simulink model "GVCU_HIL_simscape"  (R2026a)
settings: Solver=ode3  StartTime=0  StopTime=10  FixedStep=0.001
model workspace (MAT data in the model file):
  CANoelibParameters : object (value not decoded)
values from neighbouring files (symbols this model uses):
  acc_pedal_data = pedal_data.accelerator_pedal_position_t0    [Init_Simscape_main.m]
  acc_pedal_time = pedal_data.t0    [Init_Simscape_main.m]
  brk_pedal_data = brake_pedal_data.shared_brakes_drvrBrkPedlPerc_t0    [Init_Simscape_main.m]
  brk_pedal_time = brake_pedal_data.t0    [Init_Simscape_main.m]
  cycle_len = zeros(1, num_cycles)    [Init_Simscape_main.m]
  cycle_speed_matrix = zeros(max_cycle_len, num_cycles)    [Init_Simscape_main.m]
  cycle_time_matrix = zeros(max_cycle_len, num_cycles)    [Init_Simscape_main.m]
  veh_speed_data = speed_data.shared_dynamicsVso_vehVelLgt_t0    [Init_Simscape_main.m]
  veh_speed_time = speed_data.t0    [Init_Simscape_main.m]
undefined symbols (not defined in the file or in its folder): Active, aero, AuxActive, bat, brake, config, environment, FL, FL_prs_voltage, FR, FR_prs_voltage, front, pos, powertrain, rear, RL, RL_prs_voltage, RR, RR_prs_voltage, tir, veh, VGetRawValueFlag, Voltage, VT2816_1_Ch1, VT2816_1_Ch2, VT2816_1_Ch3, VT2816_1_Ch4, VT2816_3_Ch13, VT2816_3_Ch14, VT7101_1_Out2, VTS, X, Y, Z
libraries: sm_lib x358, fl_lib x272, nesl_utility x193, canoelib x127, sdl_lib x36, autolibsharedcoupling x21, autolibcoupling x9, slpidlib x7, simulink x3, autolibshareddiff x3, autolibshared x3, autolibutils x1
(part 11 of 17)

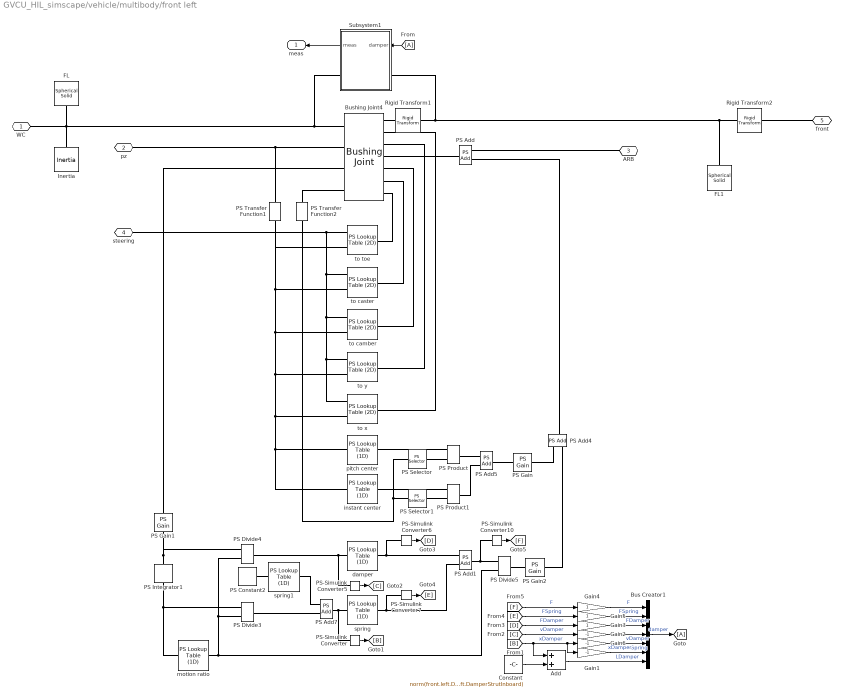
== system GVCU_HIL_simscape/vehicle/multibody/front left ==
  Add : Sum
  Bus Creator1 : BusCreator  Inputs=7
  Bushing Joint4 : sm_lib/Joints/Bushing Joint  JointMode=Normal  CompositeWrenchDir=FollowerOnBase  CompositeWrenchFrame=BaseFrame  SenseConstraintForce=off  SenseConstraintTorque=off  SenseTotalForce=on  SenseTotalTorque=off  PxPositionTargetSpecify=off  PxPositionTargetPriority=High  PxPositionTargetValue=0  PxPositionTargetValueUnits=m  PxVelocityTargetSpecify=off  PxVelocityTargetPriority=High  PxVelocityTargetValue=0  PxVelocityTargetValueUnits=m/s  PxEquilibriumPosition=0  PxEquilibriumPositionUnits=m  PxSpringStiffness=0  PxSpringStiffnessUnits=N/m  PxDampingCoefficient=0  PxDampingCoefficientUnits=N/(m/s)  PxLowerLimitSpecify=off  PxLowerLimitBound=-1  PxLowerLimitBoundUnits=m  PxLowerLimitStiffness=1e6  PxLowerLimitStiffnessUnits=N/m  PxLowerLimitDamping=1e3  PxLowerLimitDampingUnits=N/(m/s)  PxLowerLimitTransitionRegionWidth=1e-4  PxLowerLimitTransitionRegionWidthUnits=m  PxUpperLimitSpecify=off  PxUpperLimitBound=1  PxUpperLimitBoundUnits=m  PxUpperLimitStiffness=1e6  PxUpperLimitStiffnessUnits=N/m  PxUpperLimitDamping=1e3  PxUpperLimitDampingUnits=N/(m/s)  PxUpperLimitTransitionRegionWidth=1e-4  PxUpperLimitTransitionRegionWidthUnits=m  PxTorqueActuationMode=ComputedTorque  PxMotionActuationMode=InputMotion  PxSensePosition=off  PxSenseVelocity=off  PxSenseAcceleration=off  PxSenseTorqueForce=off  PxSenseLowerLimitTorqueForce=off  PxSenseUpperLimitTorqueForce=off  PyPositionTargetSpecify=off  PyPositionTargetPriority=High  PyPositionTargetValue=0  PyPositionTargetValueUnits=m  PyVelocityTargetSpecify=off  PyVelocityTargetPriority=High  PyVelocityTargetValue=0  PyVelocityTargetValueUnits=m/s  PyEquilibriumPosition=0  PyEquilibriumPositionUnits=m  PySpringStiffness=0  PySpringStiffnessUnits=N/m  PyDampingCoefficient=0  PyDampingCoefficientUnits=N/(m/s)  PyLowerLimitSpecify=off  PyLowerLimitBound=-1  PyLowerLimitBoundUnits=m  PyLowerLimitStiffness=1e6  PyLowerLimitStiffnessUnits=N/m  PyLowerLimitDamping=1e3  PyLowerLimitDampingUnits=N/(m/s)  PyLowerLimitTransitionRegionWidth=1e-4  PyLowerLimitTransitionRegionWidthUnits=m  PyUpperLimitSpecify=off  PyUpperLimitBound=1  PyUpperLimitBoundUnits=m  PyUpperLimitStiffness=1e6  PyUpperLimitStiffnessUnits=N/m  PyUpperLimitDamping=1e3  PyUpperLimitDampingUnits=N/(m/s)  PyUpperLimitTransitionRegionWidth=1e-4  PyUpperLimitTransitionRegionWidthUnits=m  PyTorqueActuationMode=ComputedTorque  PyMotionActuationMode=InputMotion  PySensePosition=off  PySenseVelocity=off  PySenseAcceleration=off  PySenseTorqueForce=off  PySenseLowerLimitTorqueForce=off  PySenseUpperLimitTorqueForce=off  PzPositionTargetSpecify=off  PzPositionTargetPriority=High  PzPositionTargetValue=0  PzPositionTargetValueUnits=m  PzVelocityTargetSpecify=off  PzVelocityTargetPriority=High  PzVelocityTargetValue=0  PzVelocityTargetValueUnits=m/s  PzEquilibriumPosition=0  PzEquilibriumPositionUnits=m  PzSpringStiffness=0  PzSpringStiffnessUnits=N/m  PzDampingCoefficient=0  PzDampingCoefficientUnits=N/(m/s)  PzLowerLimitSpecify=off  PzLowerLimitBound=-1  PzLowerLimitBoundUnits=m  PzLowerLimitStiffness=1e6  PzLowerLimitStiffnessUnits=N/m  PzLowerLimitDamping=1e3  PzLowerLimitDampingUnits=N/(m/s)  PzLowerLimitTransitionRegionWidth=1e-4  PzLowerLimitTransitionRegionWidthUnits=m  PzUpperLimitSpecify=off  PzUpperLimitBound=1  PzUpperLimitBoundUnits=m  PzUpperLimitStiffness=1e6  PzUpperLimitStiffnessUnits=N/m  PzUpperLimitDamping=1e3  PzUpperLimitDampingUnits=N/(m/s)  PzUpperLimitTransitionRegionWidth=1e-4  PzUpperLimitTransitionRegionWidthUnits=m  PzTorqueActuationMode=InputTorque  PzMotionActuationMode=ComputedMotion  PzSensePosition=on  PzSenseVelocity=on  PzSenseAcceleration=off  PzSenseTorqueForce=off  PzSenseLowerLimitTorqueForce=off  PzSenseUpperLimitTorqueForce=off  RxPositionTargetSpecify=off  RxPositionTargetPriority=High  RxPositionTargetValue=0  RxPositionTargetValueUnits=deg  RxVelocityTargetSpecify=off  RxVelocityTargetPriority=High  RxVelocityTargetValue=0  RxVelocityTargetValueUnits=deg/s  RxEquilibriumPosition=0  RxEquilibriumPositionUnits=deg  RxSpringStiffness=0  RxSpringStiffnessUnits=N*m/deg  RxDampingCoefficient=0  RxDampingCoefficientUnits=N*m/(deg/s)  RxLowerLimitSpecify=off  RxLowerLimitBound=-90  RxLowerLimitBoundUnits=deg  RxLowerLimitStiffness=1e4  RxLowerLimitStiffnessUnits=N*m/deg  RxLowerLimitDamping=10  RxLowerLimitDampingUnits=N*m/(deg/s)  RxLowerLimitTransitionRegionWidth=0.1  RxLowerLimitTransitionRegionWidthUnits=deg  RxUpperLimitSpecify=off  RxUpperLimitBound=90  RxUpperLimitBoundUnits=deg  RxUpperLimitStiffness=1e4  RxUpperLimitStiffnessUnits=N*m/deg  RxUpperLimitDamping=10  RxUpperLimitDampingUnits=N*m/(deg/s)  RxUpperLimitTransitionRegionWidth=0.1  RxUpperLimitTransitionRegionWidthUnits=deg  RxTorqueActuationMode=ComputedTorque  RxMotionActuationMode=InputMotion  RxSensePosition=off  RxSenseVelocity=off  RxSenseAcceleration=off  RxSenseTorqueForce=off  RxSenseLowerLimitTorqueForce=off  RxSenseUpperLimitTorqueForce=off  RyPositionTargetSpecify=off  RyPositionTargetPriority=High  RyPositionTargetValue=0  RyPositionTargetValueUnits=deg  RyVelocityTargetSpecify=off  RyVelocityTargetPriority=High  RyVelocityTargetValue=0  RyVelocityTargetValueUnits=deg/s  RyEquilibriumPosition=0  RyEquilibriumPositionUnits=deg  RySpringStiffness=0  RySpringStiffnessUnits=N*m/deg  RyDampingCoefficient=0  RyDampingCoefficientUnits=N*m/(deg/s)  RyLowerLimitSpecify=off  RyLowerLimitBound=-90  RyLowerLimitBoundUnits=deg  RyLowerLimitStiffness=1e4  RyLowerLimitStiffnessUnits=N*m/deg  RyLowerLimitDamping=10  RyLowerLimitDampingUnits=N*m/(deg/s)  RyLowerLimitTransitionRegionWidth=0.1  RyLowerLimitTransitionRegionWidthUnits=deg  RyUpperLimitSpecify=off  RyUpperLimitBound=90  RyUpperLimitBoundUnits=deg  RyUpperLimitStiffness=1e4  RyUpperLimitStiffnessUnits=N*m/deg  RyUpperLimitDamping=10  RyUpperLimitDampingUnits=N*m/(deg/s)  RyUpperLimitTransitionRegionWidth=0.1  RyUpperLimitTransitionRegionWidthUnits=deg  RyTorqueActuationMode=ComputedTorque  RyMotionActuationMode=InputMotion  RySensePosition=off  RySenseVelocity=off  RySenseAcceleration=off  RySenseTorqueForce=off  RySenseLowerLimitTorqueForce=off  RySenseUpperLimitTorqueForce=off  RzPositionTargetSpecify=off  RzPositionTargetPriority=High  RzPositionTargetValue=0  RzPositionTargetValueUnits=deg  RzVelocityTargetSpecify=off  RzVelocityTargetPriority=High  RzVelocityTargetValue=0  RzVelocityTargetValueUnits=deg/s  RzEquilibriumPosition=0  RzEquilibriumPositionUnits=deg  RzSpringStiffness=0  RzSpringStiffnessUnits=N*m/deg  RzDampingCoefficient=0  RzDampingCoefficientUnits=N*m/(deg/s)  RzLowerLimitSpecify=off  RzLowerLimitBound=-90  RzLowerLimitBoundUnits=deg  RzLowerLimitStiffness=1e4  RzLowerLimitStiffnessUnits=N*m/deg  RzLowerLimitDamping=10  RzLowerLimitDampingUnits=N*m/(deg/s)  RzLowerLimitTransitionRegionWidth=0.1  RzLowerLimitTransitionRegionWidthUnits=deg  RzUpperLimitSpecify=off  RzUpperLimitBound=90  RzUpperLimitBoundUnits=deg  RzUpperLimitStiffness=1e4  RzUpperLimitStiffnessUnits=N*m/deg  RzUpperLimitDamping=10  RzUpperLimitDampingUnits=N*m/(deg/s)  RzUpperLimitTransitionRegionWidth=0.1  RzUpperLimitTransitionRegionWidthUnits=deg  RzTorqueActuationMode=ComputedTorque  RzMotionActuationMode=InputMotion  RzSensePosition=off  RzSenseVelocity=off  RzSenseAcceleration=off  RzSenseTorqueForce=off  RzSenseLowerLimitTorqueForce=off  RzSenseUpperLimitTorqueForce=off
  Constant : Constant  Value=norm(front.left.DamperStrutOutboard-front.left.DamperStrutInboard)
  FL : sm_lib/Body Elements/Spherical Solid  SphereRadius=vis.joint.r  SphereRadiusUnits=m  ExportEntireGeometry=off  InertiaType=PointMass  BasedOnType=Density  Density=0  DensityUnits=kg/m^3  Mass=0  MassUnits=kg  CenterOfMass=[0 0 0]  CenterOfMassUnits=m  MomentsOfInertia=[1 1 1]  MomentsOfInertiaUnits=kg*m^2  ProductsOfInertia=[0 0 0]  ProductsOfInertiaUnits=kg*m^2  GraphicType=FromGeometry  MarkerShape=Sphere  MarkerSize=10  GraphicVisPropType=SimpleVisualProperties  GraphicDiffuseColor=vis.joint.color  GraphicOpacity=1  GraphicSpecularColor=[0.5 0.5 0.5 1.0]  GraphicAmbientColor=[0.15 0.15 0.15 1.0]  GraphicEmissiveColor=[0.0 0.0 0.0 1.0]  GraphicShininess=75  DoExposeReferenceFrame=on  SerializedFrames=<Frames/>
  FL1 : sm_lib/Body Elements/Spherical Solid  SphereRadius=vis.joint.r  SphereRadiusUnits=m  ExportEntireGeometry=off  InertiaType=PointMass  BasedOnType=Density  Density=0  DensityUnits=kg/m^3  Mass=0  MassUnits=kg  CenterOfMass=[0 0 0]  CenterOfMassUnits=m  MomentsOfInertia=[1 1 1]  MomentsOfInertiaUnits=kg*m^2  ProductsOfInertia=[0 0 0]  ProductsOfInertiaUnits=kg*m^2  GraphicType=FromGeometry  MarkerShape=Sphere  MarkerSize=10  GraphicVisPropType=SimpleVisualProperties  GraphicDiffuseColor=vis.joint.color  GraphicOpacity=1  GraphicSpecularColor=[0.5 0.5 0.5 1.0]  GraphicAmbientColor=[0.15 0.15 0.15 1.0]  GraphicEmissiveColor=[0.0 0.0 0.0 1.0]  GraphicShininess=75  DoExposeReferenceFrame=on  SerializedFrames=<Frames/>
  From : From
  Gain1 : Gain  Gain=-1
  Gain2 : Gain  Gain=-1
  Gain3 : Gain
  Gain4 : Gain
  Gain5 : Gain
  Gain6 : Gain  Gain=-1
  Goto : Goto
  Inertia : sm_lib/Body Elements/Inertia  InertiaType=PointMass  Mass=front.unsprung_mass  MassUnits=kg  CenterOfMass=[0 0 0]  CenterOfMassUnits=m  MomentsOfInertia=[1 1 1]  MomentsOfInertiaUnits=kg*m^2  ProductsOfInertia=[0 0 0]  ProductsOfInertiaUnits=kg*m^2  GraphicType=None  MarkerShape=Inertia  MarkerSize=20  GraphicVisPropType=SimpleVisualProperties  GraphicDiffuseColor=[0.5 0.5 0.5]  GraphicOpacity=1  GraphicSpecularColor=[0.5 0.5 0.5 1.0]  GraphicAmbientColor=[0.15 0.15 0.15 1.0]  GraphicEmissiveColor=[0.0 0.0 0.0 1.0]  GraphicShininess=75
  PS Add{,1,4..5,7} (5 alike) : fl_lib/Physical Signals/Functions/PS Add
  PS Constant2 : fl_lib/Physical Signals/Sources/PS Constant  constant=front.spring.preload N
  PS Divide3 : fl_lib/Physical Signals/Functions/PS Divide
  PS Divide4 : fl_lib/Physical Signals/Functions/PS Divide
  PS Divide5 : fl_lib/Physical Signals/Functions/PS Divide
  PS Gain : fl_lib/Physical Signals/Functions/PS Gain  gain=1
  PS Gain1 : fl_lib/Physical Signals/Functions/PS Gain  gain=1
  PS Gain2 : fl_lib/Physical Signals/Functions/PS Gain  gain=-1
  PS Integrator1 : fl_lib/Physical Signals/Linear Operators/PS Integrator  reset_method=foundation.enum.IntegratorResetSpec.None  initial_condition_spec=foundation.enum.IntegratorICSpec.Internal  saturation_spec=foundation.enum.IntegratorSaturationSpec.None  saturation_source_spec=foundation.enum.IntegratorSaturationSourceSpec.Internal  x0=0 m  xu=inf s  xl=-inf s
  PS Product : fl_lib/Physical Signals/Functions/PS Product
  PS Product1 : fl_lib/Physical Signals/Functions/PS Product
  PS Selector : fl_lib/Physical Signals/Nonlinear Operators/PS Selector  ix=1
  PS Selector1 : fl_lib/Physical Signals/Nonlinear Operators/PS Selector  ix=2
  PS Transfer Function1 : fl_lib/Physical Signals/Linear Operators/PS Transfer Function  transfer_function_type=foundation.enum.transfer_function_type.lag  T=0.001 s  T1=2 s  T2=1 s  reset_method=foundation.enum.IntegratorResetSpec.None  initial_condition_spec=foundation.enum.IntegratorICSpec.Internal  y0=0 m
  PS Transfer Function2 : fl_lib/Physical Signals/Linear Operators/PS Transfer Function  transfer_function_type=foundation.enum.transfer_function_type.lag  T=0.001 s  T1=2 s  T2=1 s  reset_method=foundation.enum.IntegratorResetSpec.None  initial_condition_spec=foundation.enum.IntegratorICSpec.Internal  y0=0 N
  PS-Simulink Converter{,5..7,10} (5 alike) : nesl_utility/PS-Simulink Converter  PhysicalDomain=network_engine_domain  SubClassName=ps_output  LeftPortType=input  RightPortType=output  PseudoPeriodic=off  Frequencies=[]  VectorFormat=inherit  Unit=inherit  AffineConversion=off
  Rigid Transform1 : sm_lib/Frames and Transforms/Rigid Transform  RotationMethod=RotationSequence  FollAlignAxisA=+X  BaseAlignAxisA=+Y  FollAlignAxisB=+Y  BaseAlignAxisB=+Z  RotationStandardAxis=+X  RotationAngle=0.5  RotationAngleUnits=deg  RotationArbitraryAxis=[0 0 1]  RotationSequenceAxes=FollowerAxes  RotationSequence=XYZ  RotationSequenceAngles=[-front.wheel.camber 0 front.wheel.toe]  RotationSequenceAnglesUnits=deg  RotationMatrix=[1 0 0;0 1 0;0 0 1]  Quaternion=[1 0 0 0]  TranslationMethod=None  TranslationCartesianOffset=[0 0 0]  TranslationCartesianOffsetUnits=m  TranslationStandardAxis=+Z  TranslationStandardOffset=0  TranslationStandardOffsetUnits=m  TranslationROffset=0  TranslationROffsetUnits=m  TranslationThetaOffset=0  TranslationThetaOffsetUnits=deg  TranslationZOffset=0  TranslationZOffsetUnits=m
  Rigid Transform2 : sm_lib/Frames and Transforms/Rigid Transform  RotationMethod=None  FollAlignAxisA=+X  BaseAlignAxisA=+Y  FollAlignAxisB=+Y  BaseAlignAxisB=+Z  RotationStandardAxis=+Z  RotationAngle=0  RotationAngleUnits=deg  RotationArbitraryAxis=[0 0 1]  RotationSequenceAxes=FollowerAxes  RotationSequence=XYX  RotationSequenceAngles=[0 0 0]  RotationSequenceAnglesUnits=deg  RotationMatrix=[1 0 0;0 1 0;0 0 1]  Quaternion=[1 0 0 0]  TranslationMethod=Cartesian  TranslationCartesianOffset=front.left.WheelC  TranslationCartesianOffsetUnits=m  TranslationStandardAxis=+Z  TranslationStandardOffset=0  TranslationStandardOffsetUnits=m  TranslationROffset=0  TranslationROffsetUnits=m  TranslationThetaOffset=0  TranslationThetaOffsetUnits=deg  TranslationZOffset=0  TranslationZOffsetUnits=m
  Subsystem1 : Subsystem
  damper : fl_lib/Physical Signals/Lookup Tables/PS Lookup Table (1D)  x=front.damper.v m/s  f=front.damper.N N  interp_method=simscape.enum.interpolation.linear  extrap_method=simscape.enum.extrapolation.linear
  instant center : fl_lib/Physical Signals/Lookup Tables/PS Lookup Table (1D)  x=front.z_bp m  f=tan(-front.IC_alpha)  interp_method=simscape.enum.interpolation.linear  extrap_method=simscape.enum.extrapolation.linear
  motion ratio : fl_lib/Physical Signals/Lookup Tables/PS Lookup Table (1D)  x=front.z_bp m  f=front.spring.mr_bp  interp_method=simscape.enum.interpolation.linear  extrap_method=simscape.enum.extrapolation.nearest
  pitch center : fl_lib/Physical Signals/Lookup Tables/PS Lookup Table (1D)  x=front.z_bp m  f=tan(-front.PC_alpha)  interp_method=simscape.enum.interpolation.linear  extrap_method=simscape.enum.extrapolation.linear
  spring : fl_lib/Physical Signals/Lookup Tables/PS Lookup Table (1D)  x=front.spring.l m  f=front.spring.N N  interp_method=simscape.enum.interpolation.linear  extrap_method=simscape.enum.extrapolation.linear
  spring1 : fl_lib/Physical Signals/Lookup Tables/PS Lookup Table (1D)  x=front.spring.N(2:end) N  f=front.spring.l(2:end) m  interp_method=simscape.enum.interpolation.linear  extrap_method=simscape.enum.extrapolation.linear
  to camber : fl_lib/Physical Signals/Lookup Tables/PS Lookup Table (2D)  x1=front.tierod_bp m  x2=front.z_bp m  f=front.left.camber_bp rad  interp_method=simscape.enum.interpolation.linear  extrap_method=simscape.enum.extrapolation.linear
  to caster : fl_lib/Physical Signals/Lookup Tables/PS Lookup Table (2D)  x1=front.tierod_bp m  x2=front.z_bp m  f=front.left.caster_bp rad  interp_method=simscape.enum.interpolation.linear  extrap_method=simscape.enum.extrapolation.linear
  to toe : fl_lib/Physical Signals/Lookup Tables/PS Lookup Table (2D)  x1=front.tierod_bp m  x2=front.z_bp m  f=front.left.toe_bp rad  interp_method=simscape.enum.interpolation.linear  extrap_method=simscape.enum.extrapolation.linear
  to x : fl_lib/Physical Signals/Lookup Tables/PS Lookup Table (2D)  x1=front.tierod_bp m  x2=front.z_bp m  f=front.left.x_bp m  interp_method=simscape.enum.interpolation.linear  extrap_method=simscape.enum.extrapolation.linear
  to y : fl_lib/Physical Signals/Lookup Tables/PS Lookup Table (2D)  x1=front.tierod_bp m  x2=front.z_bp m  f=front.left.y_bp m  interp_method=simscape.enum.interpolation.linear  extrap_method=simscape.enum.extrapolation.linear
  WC : PMIOPort  Side=Left
  pz : PMIOPort  Port=2  Side=Right
  ARB : PMIOPort  Port=3  Side=Right
  steering : PMIOPort  Port=4  Side=Right
  front : PMIOPort  Port=5  Side=Right
  meas : Outport
  wires:
  Subsystem1/1(meas) -> meas/1
  Add/1 -> Bus Creator1/7  "LDamper"
  Bus Creator1/1 -> Goto/1  "damper"
  [E] -> Gain5/1  "FSpring"
  Gain2/1 -> Bus Creator1/4  "vDamper"
  Gain1/1 -> Bus Creator1/6  "xSpring"
  [D] -> Gain3/1  "FDamper"
  Gain4/1 -> Bus Creator1/1  "F"
  [C] -> Gain2/1  "vDamper"
  [F] -> Gain4/1  "F"
  Gain3/1 -> Bus Creator1/3  "FDamper"
  Gain6/1 -> Bus Creator1/5  "xDamper"
  Gain5/1 -> Bus Creator1/2  "FSpring"
  [B] -> Add/1, Gain1/1, Gain6/1  "xDamper"
  From/1 -> Subsystem1/1(damper)
  PS-Simulink Converter5/1 -> [C]
  PS-Simulink Converter6/1 -> [D]
  PS-Simulink Converter7/1 -> [E]
  PS-Simulink Converter10/1 -> [F]
  Constant/1 -> Add/2
  PS-Simulink Converter/1 -> [B]
  connections:
  Bushing Joint4/RConn1 -- Subsystem1/RConn1 -- FL/RConn1 -- WC/RConn1 -- Inertia/RConn1
  Subsystem1/LConn1 -- Rigid Transform1/LConn1 -- Rigid Transform2/RConn1 -- FL1/RConn1
  front/RConn1 -- Rigid Transform2/LConn1
  instant center/LConn1 -- pitch center/LConn1 -- to x/LConn2 -- to y/LConn2 -- to camber/LConn2 -- to caster/LConn2 -- PS Transfer Function1/RConn1 -- to toe/LConn2
  to x/RConn1 -- Bushing Joint4/LConn2
  to y/RConn1 -- Bushing Joint4/LConn3
  to caster/RConn1 -- Bushing Joint4/LConn6
  PS Gain1/LConn1 -- Bushing Joint4/RConn3
  PS Add/RConn1 -- Bushing Joint4/LConn4
  ARB/RConn1 -- PS Add/LConn2
  to x/LConn1 -- to y/LConn1 -- to camber/LConn1 -- to caster/LConn1 -- steering/RConn1 -- to toe/LConn1
  Bushing Joint4/RConn2 -- PS Transfer Function1/LConn1 -- pz/RConn1
  to toe/RConn1 -- Bushing Joint4/LConn7
  to camber/RConn1 -- Bushing Joint4/LConn5
  Bushing Joint4/LConn1 -- Rigid Transform1/RConn1
  PS Divide5/LConn1 -- PS-Simulink Converter10/LConn1 -- PS Add1/RConn1
  motion ratio/LConn1 -- PS Integrator1/RConn1 -- PS Divide3/LConn1
  PS Divide4/LConn2 -- PS Divide3/LConn2 -- PS Divide5/LConn2 -- motion ratio/RConn1
  PS Integrator1/LConn1 -- PS Divide4/LConn1 -- PS Gain1/RConn1
  PS Divide4/RConn1 -- PS-Simulink Converter5/LConn1 -- damper/LConn1
  PS Add1/LConn1 -- PS-Simulink Converter6/LConn1 -- damper/RConn1
  PS Gain2/LConn1 -- PS Divide5/RConn1
  PS Add4/RConn1 -- PS Add/LConn1
  PS Transfer Function2/LConn1 -- Bushing Joint4/RConn4
  PS Selector/LConn1 -- PS Selector1/LConn1 -- PS Transfer Function2/RConn1
  PS Selector/RConn1 -- PS Product/LConn2
  pitch center/RConn1 -- PS Product/LConn1
  PS Selector1/RConn1 -- PS Product1/LConn2
  instant center/RConn1 -- PS Product1/LConn1
  PS Gain/RConn1 -- PS Add4/LConn1
  PS Add5/RConn1 -- PS Gain/LConn1
  PS Add5/LConn1 -- PS Product/RConn1
  PS Product1/RConn1 -- PS Add5/LConn2
  PS Gain2/RConn1 -- PS Add4/LConn2
  spring1/RConn1 -- PS Add7/LConn1
  spring/RConn1 -- PS Add1/LConn2 -- PS-Simulink Converter7/LConn1
  PS Add7/RConn1 -- PS-Simulink Converter/LConn1 -- spring/LConn1
  spring1/LConn1 -- PS Constant2/RConn1
  PS Divide3/RConn1 -- PS Add7/LConn2

== system GVCU_HIL_simscape/vehicle/multibody/front left contact ==
  friction : Inport
  Bus Creator : BusCreator  Inputs=12
  Bus Selector : BusSelector  OutputSignals=front_left_lmux,front_left_lmuy
  Infinite Plane1 : sm_lib/Curves and Surfaces/Infinite Plane  GraphicType=None  GraphicPlaneWidth=1  GraphicPlaneWidthUnits=m  GraphicPlaneHeight=1  GraphicPlaneHeightUnits=m  GraphicVisPropType=SimpleVisualProperties  GraphicDiffuseColor=[0.5 0.5 0.5]  GraphicOpacity=0.1  GraphicSpecularColor=[0.5 0.5 0.5 1.0]  GraphicAmbientColor=[0.15 0.15 0.15 1.0]  GraphicEmissiveColor=[0.0 0.0 0.0 1.0]  GraphicShininess=75
  Magic Formula Tire Force and Torque2 : sm_lib/Forces and Torques/Magic Formula Tire Force and Torque  TireSide=Left  TireParameters=front.wheel.magic_param  SlipMode=Combined  ContactFrameMethod=ClosestPoint  ScalingCoefficientLMUXMode=ProvidedByInput  ScalingCoefficientLMUYMode=ProvidedByInput  SenseContactSignal=off  TireWrenchFrame=ContactFrame  SenseTireForce=on  SenseTireTorque=on  SensePneumaticTrail=on  SenseLongitudinalSlip=on  SenseSaturatedLongitudinalSlip=off  SenseSlipAngle=on  SenseSaturatedSlipAngle=off  SenseTurnSlip=off  SenseRelativeLongitudinalVelocity=off  SenseRelativeLateralVelocity=off  SenseLongitudinalSlipVelocity=off  SenseLateralSlipVelocity=off  SenseYawVelocity=off  SenseCamberAngle=on  SenseSaturatedCamberAngle=off  SenseCamberVelocity=off  SenseSpinVelocity=on  SenseFreeRadius=on  SenseLoadedRadius=on  SenseEffectiveRollingRadius=on  SenseRadialDeflection=off  SenseLongitudinalFrictionCoefficient=on  SenseLateralFrictionCoefficient=on  SenseContactBaseRotation=off  SenseContactBaseTranslation=off  SenseContactFollowerRotation=off  SenseContactFollowerTranslation=off  NumericParameters=[0.1 0.1 0.1 0.1 5.0 1e-4 1e-4 1e-7 1e-7 1e-4 1e-4 0.1 1e-4 1e-4 1e-4 1e-4 1e-4 1e-4 1e-4 1e-4 1e-4]
  Mechanical Rotational Reference : fl_lib/Mechanical/Rotational Elements/Mechanical Rotational Reference
  PS-Simulink Converter{,1..11} (12 alike) : nesl_utility/PS-Simulink Converter  PhysicalDomain=network_engine_domain  SubClassName=ps_output  LeftPortType=input  RightPortType=output  PseudoPeriodic=off  Frequencies=[]  VectorFormat=inherit  Unit=inherit  AffineConversion=off
  Revolute Joint : sm_lib/Joints/Revolute Joint  JointMode=Normal  CompositeWrenchDir=FollowerOnBase  CompositeWrenchFrame=BaseFrame  SenseConstraintForce=off  SenseConstraintTorque=off  SenseTotalForce=off  SenseTotalTorque=off  PositionTargetSpecify=off  PositionTargetPriority=High  PositionTargetValue=0  PositionTargetValueUnits=deg  VelocityTargetSpecify=off  VelocityTargetPriority=High  VelocityTargetValue=0  VelocityTargetValueUnits=deg/s  EquilibriumPosition=0  EquilibriumPositionUnits=deg  SpringStiffness=0  SpringStiffnessUnits=N*m/deg  DampingCoefficient=0  DampingCoefficientUnits=N*m/(deg/s)  LowerLimitSpecify=off  LowerLimitBound=-90  LowerLimitBoundUnits=deg  LowerLimitStiffness=1e4  LowerLimitStiffnessUnits=N*m/deg  LowerLimitDamping=10  LowerLimitDampingUnits=N*m/(deg/s)  LowerLimitTransitionRegionWidth=0.1  LowerLimitTransitionRegionWidthUnits=deg  UpperLimitSpecify=off  UpperLimitBound=90  UpperLimitBoundUnits=deg  UpperLimitStiffness=1e4  UpperLimitStiffnessUnits=N*m/deg  UpperLimitDamping=10  UpperLimitDampingUnits=N*m/(deg/s)  UpperLimitTransitionRegionWidth=0.1  UpperLimitTransitionRegionWidthUnits=deg  TorqueActuationMode=InputTorque  MotionActuationMode=ComputedMotion  SensePosition=off  SenseVelocity=on  SenseAcceleration=off  SenseTorqueForce=off  SenseLowerLimitTorqueForce=off  SenseUpperLimitTorqueForce=off
  Rigid Transform4 : sm_lib/Frames and Transforms/Rigid Transform  RotationMethod=StandardAxis  FollAlignAxisA=+X  BaseAlignAxisA=+Y  FollAlignAxisB=+Y  BaseAlignAxisB=+Z  RotationStandardAxis=-X  RotationAngle=90  RotationAngleUnits=deg  RotationArbitraryAxis=[0 0 1]  RotationSequenceAxes=FollowerAxes  RotationSequence=XYX  RotationSequenceAngles=[0 0 0]  RotationSequenceAnglesUnits=deg  RotationMatrix=[1 0 0;0 1 0;0 0 1]  Quaternion=[1 0 0 0]  TranslationMethod=None  TranslationCartesianOffset=[0 0 0]  TranslationCartesianOffsetUnits=m  TranslationStandardAxis=+Z  TranslationStandardOffset=0  TranslationStandardOffsetUnits=m  TranslationROffset=0  TranslationROffsetUnits=m  TranslationThetaOffset=0  TranslationThetaOffsetUnits=deg  TranslationZOffset=0  TranslationZOffsetUnits=m
  Rotational Multibody Interface : fl_lib/Mechanical/Multibody Interfaces/Rotational Multibody Interface
  Simulink-PS Converter : nesl_utility/Simulink-PS Converter  PhysicalDomain=network_engine_domain  SubClassName=ps_input  LeftPortType=input  RightPortType=output  PseudoPeriodic=off  Frequencies=[]  NoiseDistribution=none  NoiseParameters=[]  Unit=1  AffineConversion=off  FilteringAndDerivatives=provide  SimscapeFilterOrder=1  InputFilterTimeConstant=0.001  UdotUserProvided=0
  Simulink-PS Converter1 : nesl_utility/Simulink-PS Converter  PhysicalDomain=network_engine_domain  SubClassName=ps_input  LeftPortType=input  RightPortType=output  PseudoPeriodic=off  Frequencies=[]  NoiseDistribution=none  NoiseParameters=[]  Unit=1  AffineConversion=off  FilteringAndDerivatives=provide  SimscapeFilterOrder=1  InputFilterTimeConstant=0.001  UdotUserProvided=0
  World Frame : sm_lib/Frames and Transforms/World Frame
  wheel : Subsystem
      settings: PortSchema="{\"entries\":[{\"content\":{\"sides\":[{\"content\":{},\"type\":\"ConnectorPlacement.EquallySpacedRectSide\",\"uuid\":\"adeeef9f-292b-4510-8562-bbfd5584739c\"},{\"content\":{\"side\":\"RIGHT\"},\"type\":\"ConnectorPlacement.EquallySpacedRectSide\",\"uuid\":\"ec27151e-0c19-490a-9fed-68b4fab3fecb\"},{\"content\":{\"side\":\"TOP\"},\"type\":\"ConnectorPlacement.EquallySpacedRectSide\",\"uuid\":\"2927d071-59e0-4510-913d-c0d529befb9e\"},{\"content\":{\"connectorIds\":[\"RConn1\"],\"side\":\"BOTTOM\"},\"type\":\"ConnectorPlacement.EquallySpacedRectSide\",\"uuid\":\"52ecb1bf-4068-4c10-840d-d5f54d46844d\"}]},\"type\":\"ConnectorPlacement.EquallySpacedConnector\",\"uuid\":\"677d5654-c51c-421b-8b5c-9ce4476cb5a7\"}],\"packageUris\":[\"http://schema.mathworks.com/mf0/Connector/R2020b\"],\"version\":\"1.0\"}"
  WC : PMIOPort  Side=Right
  trq : PMIOPort  Port=2  Side=Right
  meas : Outport
  wires:
  PS-Simulink Converter7/1 -> Bus Creator/11  "mux"
  PS-Simulink Converter2/1 -> Bus Creator/5  "alpha"
  PS-Simulink Converter/1 -> Bus Creator/2  "T"
  PS-Simulink Converter1/1 -> Bus Creator/4  "kappa"
  PS-Simulink Converter8/1 -> Bus Creator/1  "F"
  PS-Simulink Converter4/1 -> Bus Creator/8  "free_radius"
  PS-Simulink Converter3/1 -> Bus Creator/6  "gamma"
  PS-Simulink Converter5/1 -> Bus Creator/9  "loaded_radius"
  PS-Simulink Converter6/1 -> Bus Creator/10  "eff_roll_radius"
  Bus Creator/1 -> meas/1  "tire"
  PS-Simulink Converter10/1 -> Bus Creator/7  "omega"
  PS-Simulink Converter9/1 -> Bus Creator/12  "muy"
  PS-Simulink Converter11/1 -> Bus Creator/3  "p_trail"
  friction/1 -> Bus Selector/1
  Bus Selector/1 -> Simulink-PS Converter/1  "<front_left_lmux>"
  Bus Selector/2 -> Simulink-PS Converter1/1  "<front_left_lmuy>"
  connections:
  Magic Formula Tire Force and Torque2/RConn7 -- PS-Simulink Converter3/LConn1
  Magic Formula Tire Force and Torque2/RConn4 -- PS-Simulink Converter11/LConn1
  Magic Formula Tire Force and Torque2/RConn11 -- PS-Simulink Converter6/LConn1
  WC/RConn1 -- Rigid Transform4/LConn1
  Magic Formula Tire Force and Torque2/RConn2 -- PS-Simulink Converter8/LConn1
  Magic Formula Tire Force and Torque2/RConn8 -- PS-Simulink Converter10/LConn1
  Magic Formula Tire Force and Torque2/RConn10 -- PS-Simulink Converter5/LConn1
  Revolute Joint/RConn1 -- Magic Formula Tire Force and Torque2/RConn1 -- wheel/RConn1
  Magic Formula Tire Force and Torque2/RConn6 -- PS-Simulink Converter2/LConn1
  Magic Formula Tire Force and Torque2/RConn5 -- PS-Simulink Converter1/LConn1
  Magic Formula Tire Force and Torque2/RConn12 -- PS-Simulink Converter7/LConn1
  Magic Formula Tire Force and Torque2/RConn3 -- PS-Simulink Converter/LConn1
  Rigid Transform4/RConn1 -- Revolute Joint/LConn1
  Magic Formula Tire Force and Torque2/RConn9 -- PS-Simulink Converter4/LConn1
  Revolute Joint/RConn2 -- Rotational Multibody Interface/RConn1
  Rotational Multibody Interface/LConn1 -- Revolute Joint/LConn2
  Mechanical Rotational Reference/LConn1 -- Rotational Multibody Interface/LConn2
  trq/RConn1 -- Rotational Multibody Interface/RConn2
  Infinite Plane1/RConn1 -- Magic Formula Tire Force and Torque2/LConn1
  Infinite Plane1/LConn1 -- World Frame/RConn1
  Magic Formula Tire Force and Torque2/RConn13 -- PS-Simulink Converter9/LConn1
  Simulink-PS Converter/RConn1 -- Magic Formula Tire Force and Torque2/LConn2
  Simulink-PS Converter1/RConn1 -- Magic Formula Tire Force and Torque2/LConn3

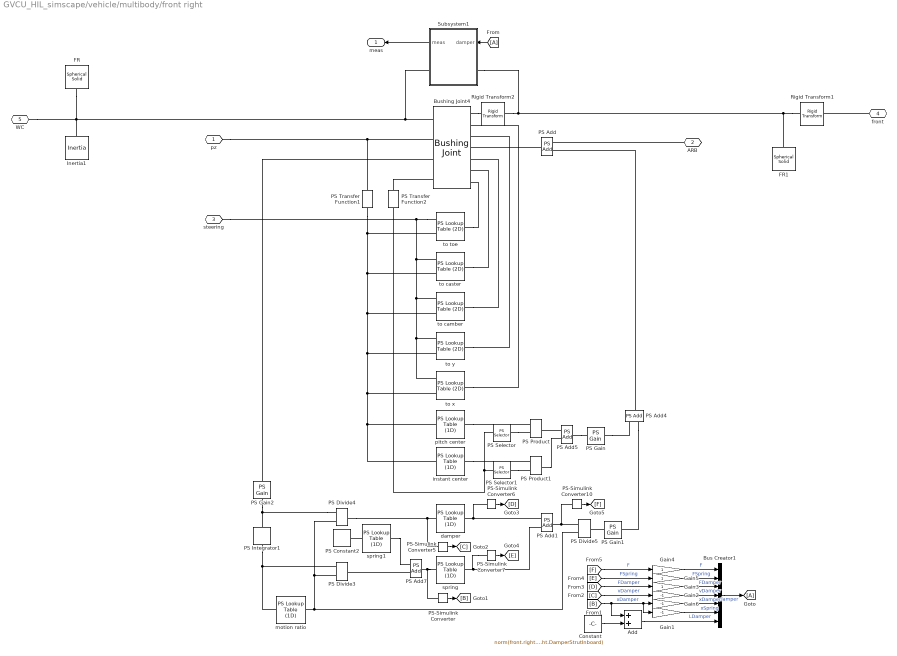
== system GVCU_HIL_simscape/vehicle/multibody/front right ==
  Add : Sum
  Bus Creator1 : BusCreator  Inputs=7
  Bushing Joint4 : sm_lib/Joints/Bushing Joint  JointMode=Normal  CompositeWrenchDir=FollowerOnBase  CompositeWrenchFrame=BaseFrame  SenseConstraintForce=off  SenseConstraintTorque=off  SenseTotalForce=on  SenseTotalTorque=off  PxPositionTargetSpecify=off  PxPositionTargetPriority=High  PxPositionTargetValue=0  PxPositionTargetValueUnits=m  PxVelocityTargetSpecify=off  PxVelocityTargetPriority=High  PxVelocityTargetValue=0  PxVelocityTargetValueUnits=m/s  PxEquilibriumPosition=0  PxEquilibriumPositionUnits=m  PxSpringStiffness=0  PxSpringStiffnessUnits=N/m  PxDampingCoefficient=0  PxDampingCoefficientUnits=N/(m/s)  PxLowerLimitSpecify=off  PxLowerLimitBound=-1  PxLowerLimitBoundUnits=m  PxLowerLimitStiffness=1e6  PxLowerLimitStiffnessUnits=N/m  PxLowerLimitDamping=1e3  PxLowerLimitDampingUnits=N/(m/s)  PxLowerLimitTransitionRegionWidth=1e-4  PxLowerLimitTransitionRegionWidthUnits=m  PxUpperLimitSpecify=off  PxUpperLimitBound=1  PxUpperLimitBoundUnits=m  PxUpperLimitStiffness=1e6  PxUpperLimitStiffnessUnits=N/m  PxUpperLimitDamping=1e3  PxUpperLimitDampingUnits=N/(m/s)  PxUpperLimitTransitionRegionWidth=1e-4  PxUpperLimitTransitionRegionWidthUnits=m  PxTorqueActuationMode=ComputedTorque  PxMotionActuationMode=InputMotion  PxSensePosition=off  PxSenseVelocity=off  PxSenseAcceleration=off  PxSenseTorqueForce=off  PxSenseLowerLimitTorqueForce=off  PxSenseUpperLimitTorqueForce=off  PyPositionTargetSpecify=off  PyPositionTargetPriority=High  PyPositionTargetValue=0  PyPositionTargetValueUnits=m  PyVelocityTargetSpecify=off  PyVelocityTargetPriority=High  PyVelocityTargetValue=0  PyVelocityTargetValueUnits=m/s  PyEquilibriumPosition=0  PyEquilibriumPositionUnits=m  PySpringStiffness=0  PySpringStiffnessUnits=N/m  PyDampingCoefficient=0  PyDampingCoefficientUnits=N/(m/s)  PyLowerLimitSpecify=off  PyLowerLimitBound=-1  PyLowerLimitBoundUnits=m  PyLowerLimitStiffness=1e6  PyLowerLimitStiffnessUnits=N/m  PyLowerLimitDamping=1e3  PyLowerLimitDampingUnits=N/(m/s)  PyLowerLimitTransitionRegionWidth=1e-4  PyLowerLimitTransitionRegionWidthUnits=m  PyUpperLimitSpecify=off  PyUpperLimitBound=1  PyUpperLimitBoundUnits=m  PyUpperLimitStiffness=1e6  PyUpperLimitStiffnessUnits=N/m  PyUpperLimitDamping=1e3  PyUpperLimitDampingUnits=N/(m/s)  PyUpperLimitTransitionRegionWidth=1e-4  PyUpperLimitTransitionRegionWidthUnits=m  PyTorqueActuationMode=ComputedTorque  PyMotionActuationMode=InputMotion  PySensePosition=off  PySenseVelocity=off  PySenseAcceleration=off  PySenseTorqueForce=off  PySenseLowerLimitTorqueForce=off  PySenseUpperLimitTorqueForce=off  PzPositionTargetSpecify=off  PzPositionTargetPriority=High  PzPositionTargetValue=0  PzPositionTargetValueUnits=m  PzVelocityTargetSpecify=off  PzVelocityTargetPriority=High  PzVelocityTargetValue=0  PzVelocityTargetValueUnits=m/s  PzEquilibriumPosition=0  PzEquilibriumPositionUnits=m  PzSpringStiffness=0  PzSpringStiffnessUnits=N/m  PzDampingCoefficient=0  PzDampingCoefficientUnits=N/(m/s)  PzLowerLimitSpecify=off  PzLowerLimitBound=-1  PzLowerLimitBoundUnits=m  PzLowerLimitStiffness=1e6  PzLowerLimitStiffnessUnits=N/m  PzLowerLimitDamping=1e3  PzLowerLimitDampingUnits=N/(m/s)  PzLowerLimitTransitionRegionWidth=1e-4  PzLowerLimitTransitionRegionWidthUnits=m  PzUpperLimitSpecify=off  PzUpperLimitBound=1  PzUpperLimitBoundUnits=m  PzUpperLimitStiffness=1e6  PzUpperLimitStiffnessUnits=N/m  PzUpperLimitDamping=1e3  PzUpperLimitDampingUnits=N/(m/s)  PzUpperLimitTransitionRegionWidth=1e-4  PzUpperLimitTransitionRegionWidthUnits=m  PzTorqueActuationMode=InputTorque  PzMotionActuationMode=ComputedMotion  PzSensePosition=on  PzSenseVelocity=on  PzSenseAcceleration=off  PzSenseTorqueForce=off  PzSenseLowerLimitTorqueForce=off  PzSenseUpperLimitTorqueForce=off  RxPositionTargetSpecify=off  RxPositionTargetPriority=High  RxPositionTargetValue=0  RxPositionTargetValueUnits=deg  RxVelocityTargetSpecify=off  RxVelocityTargetPriority=High  RxVelocityTargetValue=0  RxVelocityTargetValueUnits=deg/s  RxEquilibriumPosition=0  RxEquilibriumPositionUnits=deg  RxSpringStiffness=0  RxSpringStiffnessUnits=N*m/deg  RxDampingCoefficient=0  RxDampingCoefficientUnits=N*m/(deg/s)  RxLowerLimitSpecify=off  RxLowerLimitBound=-90  RxLowerLimitBoundUnits=deg  RxLowerLimitStiffness=1e4  RxLowerLimitStiffnessUnits=N*m/deg  RxLowerLimitDamping=10  RxLowerLimitDampingUnits=N*m/(deg/s)  RxLowerLimitTransitionRegionWidth=0.1  RxLowerLimitTransitionRegionWidthUnits=deg  RxUpperLimitSpecify=off  RxUpperLimitBound=90  RxUpperLimitBoundUnits=deg  RxUpperLimitStiffness=1e4  RxUpperLimitStiffnessUnits=N*m/deg  RxUpperLimitDamping=10  RxUpperLimitDampingUnits=N*m/(deg/s)  RxUpperLimitTransitionRegionWidth=0.1  RxUpperLimitTransitionRegionWidthUnits=deg  RxTorqueActuationMode=ComputedTorque  RxMotionActuationMode=InputMotion  RxSensePosition=off  RxSenseVelocity=off  RxSenseAcceleration=off  RxSenseTorqueForce=off  RxSenseLowerLimitTorqueForce=off  RxSenseUpperLimitTorqueForce=off  RyPositionTargetSpecify=off  RyPositionTargetPriority=High  RyPositionTargetValue=0  RyPositionTargetValueUnits=deg  RyVelocityTargetSpecify=off  RyVelocityTargetPriority=High  RyVelocityTargetValue=0  RyVelocityTargetValueUnits=deg/s  RyEquilibriumPosition=0  RyEquilibriumPositionUnits=deg  RySpringStiffness=0  RySpringStiffnessUnits=N*m/deg  RyDampingCoefficient=0  RyDampingCoefficientUnits=N*m/(deg/s)  RyLowerLimitSpecify=off  RyLowerLimitBound=-90  RyLowerLimitBoundUnits=deg  RyLowerLimitStiffness=1e4  RyLowerLimitStiffnessUnits=N*m/deg  RyLowerLimitDamping=10  RyLowerLimitDampingUnits=N*m/(deg/s)  RyLowerLimitTransitionRegionWidth=0.1  RyLowerLimitTransitionRegionWidthUnits=deg  RyUpperLimitSpecify=off  RyUpperLimitBound=90  RyUpperLimitBoundUnits=deg  RyUpperLimitStiffness=1e4  RyUpperLimitStiffnessUnits=N*m/deg  RyUpperLimitDamping=10  RyUpperLimitDampingUnits=N*m/(deg/s)  RyUpperLimitTransitionRegionWidth=0.1  RyUpperLimitTransitionRegionWidthUnits=deg  RyTorqueActuationMode=ComputedTorque  RyMotionActuationMode=InputMotion  RySensePosition=off  RySenseVelocity=off  RySenseAcceleration=off  RySenseTorqueForce=off  RySenseLowerLimitTorqueForce=off  RySenseUpperLimitTorqueForce=off  RzPositionTargetSpecify=off  RzPositionTargetPriority=High  RzPositionTargetValue=0  RzPositionTargetValueUnits=deg  RzVelocityTargetSpecify=off  RzVelocityTargetPriority=High  RzVelocityTargetValue=0  RzVelocityTargetValueUnits=deg/s  RzEquilibriumPosition=0  RzEquilibriumPositionUnits=deg  RzSpringStiffness=0  RzSpringStiffnessUnits=N*m/deg  RzDampingCoefficient=0  RzDampingCoefficientUnits=N*m/(deg/s)  RzLowerLimitSpecify=off  RzLowerLimitBound=-90  RzLowerLimitBoundUnits=deg  RzLowerLimitStiffness=1e4  RzLowerLimitStiffnessUnits=N*m/deg  RzLowerLimitDamping=10  RzLowerLimitDampingUnits=N*m/(deg/s)  RzLowerLimitTransitionRegionWidth=0.1  RzLowerLimitTransitionRegionWidthUnits=deg  RzUpperLimitSpecify=off  RzUpperLimitBound=90  RzUpperLimitBoundUnits=deg  RzUpperLimitStiffness=1e4  RzUpperLimitStiffnessUnits=N*m/deg  RzUpperLimitDamping=10  RzUpperLimitDampingUnits=N*m/(deg/s)  RzUpperLimitTransitionRegionWidth=0.1  RzUpperLimitTransitionRegionWidthUnits=deg  RzTorqueActuationMode=ComputedTorque  RzMotionActuationMode=InputMotion  RzSensePosition=off  RzSenseVelocity=off  RzSenseAcceleration=off  RzSenseTorqueForce=off  RzSenseLowerLimitTorqueForce=off  RzSenseUpperLimitTorqueForce=off
  Constant : Constant  Value=norm(front.right.DamperStrutOutboard-front.right.DamperStrutInboard)
  FR : sm_lib/Body Elements/Spherical Solid  SphereRadius=vis.joint.r  SphereRadiusUnits=m  ExportEntireGeometry=off  InertiaType=PointMass  BasedOnType=Density  Density=0  DensityUnits=kg/m^3  Mass=0  MassUnits=kg  CenterOfMass=[0 0 0]  CenterOfMassUnits=m  MomentsOfInertia=[1 1 1]  MomentsOfInertiaUnits=kg*m^2  ProductsOfInertia=[0 0 0]  ProductsOfInertiaUnits=kg*m^2  GraphicType=FromGeometry  MarkerShape=Sphere  MarkerSize=10  GraphicVisPropType=SimpleVisualProperties  GraphicDiffuseColor=vis.joint.color  GraphicOpacity=1  GraphicSpecularColor=[0.5 0.5 0.5 1.0]  GraphicAmbientColor=[0.15 0.15 0.15 1.0]  GraphicEmissiveColor=[0.0 0.0 0.0 1.0]  GraphicShininess=75  DoExposeReferenceFrame=on  SerializedFrames=<Frames/>
  FR1 : sm_lib/Body Elements/Spherical Solid  SphereRadius=vis.joint.r  SphereRadiusUnits=m  ExportEntireGeometry=off  InertiaType=PointMass  BasedOnType=Density  Density=0  DensityUnits=kg/m^3  Mass=0  MassUnits=kg  CenterOfMass=[0 0 0]  CenterOfMassUnits=m  MomentsOfInertia=[1 1 1]  MomentsOfInertiaUnits=kg*m^2  ProductsOfInertia=[0 0 0]  ProductsOfInertiaUnits=kg*m^2  GraphicType=FromGeometry  MarkerShape=Sphere  MarkerSize=10  GraphicVisPropType=SimpleVisualProperties  GraphicDiffuseColor=vis.joint.color  GraphicOpacity=1  GraphicSpecularColor=[0.5 0.5 0.5 1.0]  GraphicAmbientColor=[0.15 0.15 0.15 1.0]  GraphicEmissiveColor=[0.0 0.0 0.0 1.0]  GraphicShininess=75  DoExposeReferenceFrame=on  SerializedFrames=<Frames/>
  From : From
  Gain1 : Gain  Gain=-1
  Gain2 : Gain  Gain=-1
  Gain3 : Gain
  Gain4 : Gain
  Gain5 : Gain
  Gain6 : Gain  Gain=-1
  Goto : Goto
  Inertia1 : sm_lib/Body Elements/Inertia  InertiaType=PointMass  Mass=front.unsprung_mass  MassUnits=kg  CenterOfMass=[0 0 0]  CenterOfMassUnits=m  MomentsOfInertia=[1 1 1]  MomentsOfInertiaUnits=kg*m^2  ProductsOfInertia=[0 0 0]  ProductsOfInertiaUnits=kg*m^2  GraphicType=None  MarkerShape=Inertia  MarkerSize=20  GraphicVisPropType=SimpleVisualProperties  GraphicDiffuseColor=[0.5 0.5 0.5]  GraphicOpacity=1  GraphicSpecularColor=[0.5 0.5 0.5 1.0]  GraphicAmbientColor=[0.15 0.15 0.15 1.0]  GraphicEmissiveColor=[0.0 0.0 0.0 1.0]  GraphicShininess=75
  PS Add{,1,4..5,7} (5 alike) : fl_lib/Physical Signals/Functions/PS Add
  PS Constant2 : fl_lib/Physical Signals/Sources/PS Constant  constant=front.spring.preload N
  PS Divide3 : fl_lib/Physical Signals/Functions/PS Divide
  PS Divide4 : fl_lib/Physical Signals/Functions/PS Divide
  PS Divide5 : fl_lib/Physical Signals/Functions/PS Divide
  PS Gain : fl_lib/Physical Signals/Functions/PS Gain  gain=1
  PS Gain1 : fl_lib/Physical Signals/Functions/PS Gain  gain=-1
  PS Gain2 : fl_lib/Physical Signals/Functions/PS Gain  gain=1
  PS Integrator1 : fl_lib/Physical Signals/Linear Operators/PS Integrator  reset_method=foundation.enum.IntegratorResetSpec.None  initial_condition_spec=foundation.enum.IntegratorICSpec.Internal  saturation_spec=foundation.enum.IntegratorSaturationSpec.None  saturation_source_spec=foundation.enum.IntegratorSaturationSourceSpec.Internal  x0=0 m  xu=inf s  xl=-inf s
  PS Product : fl_lib/Physical Signals/Functions/PS Product
  PS Product1 : fl_lib/Physical Signals/Functions/PS Product
  PS Selector : fl_lib/Physical Signals/Nonlinear Operators/PS Selector  ix=1
  PS Selector1 : fl_lib/Physical Signals/Nonlinear Operators/PS Selector  ix=2
  PS Transfer Function1 : fl_lib/Physical Signals/Linear Operators/PS Transfer Function  transfer_function_type=foundation.enum.transfer_function_type.lag  T=0.001 s  T1=2 s  T2=1 s  reset_method=foundation.enum.IntegratorResetSpec.None  initial_condition_spec=foundation.enum.IntegratorICSpec.Internal  y0=0 m
  PS Transfer Function2 : fl_lib/Physical Signals/Linear Operators/PS Transfer Function  transfer_function_type=foundation.enum.transfer_function_type.lag  T=0.001 s  T1=2 s  T2=1 s  reset_method=foundation.enum.IntegratorResetSpec.None  initial_condition_spec=foundation.enum.IntegratorICSpec.Internal  y0=0 N
  PS-Simulink Converter{,5..7,10} (5 alike) : nesl_utility/PS-Simulink Converter  PhysicalDomain=network_engine_domain  SubClassName=ps_output  LeftPortType=input  RightPortType=output  PseudoPeriodic=off  Frequencies=[]  VectorFormat=inherit  Unit=inherit  AffineConversion=off
  Rigid Transform1 : sm_lib/Frames and Transforms/Rigid Transform  RotationMethod=None  FollAlignAxisA=+X  BaseAlignAxisA=+Y  FollAlignAxisB=+Y  BaseAlignAxisB=+Z  RotationStandardAxis=+Z  RotationAngle=0  RotationAngleUnits=deg  RotationArbitraryAxis=[0 0 1]  RotationSequenceAxes=FollowerAxes  RotationSequence=XYX  RotationSequenceAngles=[0 0 0]  RotationSequenceAnglesUnits=deg  RotationMatrix=[1 0 0;0 1 0;0 0 1]  Quaternion=[1 0 0 0]  TranslationMethod=Cartesian  TranslationCartesianOffset=front.right.WheelC  TranslationCartesianOffsetUnits=m  TranslationStandardAxis=+Z  TranslationStandardOffset=0  TranslationStandardOffsetUnits=m  TranslationROffset=0  TranslationROffsetUnits=m  TranslationThetaOffset=0  TranslationThetaOffsetUnits=deg  TranslationZOffset=0  TranslationZOffsetUnits=m
  Rigid Transform2 : sm_lib/Frames and Transforms/Rigid Transform  RotationMethod=RotationSequence  FollAlignAxisA=+X  BaseAlignAxisA=+Y  FollAlignAxisB=+Y  BaseAlignAxisB=+Z  RotationStandardAxis=+X  RotationAngle=0.5  RotationAngleUnits=deg  RotationArbitraryAxis=[0 0 1]  RotationSequenceAxes=FollowerAxes  RotationSequence=XYZ  RotationSequenceAngles=[front.wheel.camber 0 -front.wheel.toe]  RotationSequenceAnglesUnits=deg  RotationMatrix=[1 0 0;0 1 0;0 0 1]  Quaternion=[1 0 0 0]  TranslationMethod=None  TranslationCartesianOffset=[0 0 0]  TranslationCartesianOffsetUnits=m  TranslationStandardAxis=+Z  TranslationStandardOffset=0  TranslationStandardOffsetUnits=m  TranslationROffset=0  TranslationROffsetUnits=m  TranslationThetaOffset=0  TranslationThetaOffsetUnits=deg  TranslationZOffset=0  TranslationZOffsetUnits=m
  Subsystem1 : Subsystem
  damper : fl_lib/Physical Signals/Lookup Tables/PS Lookup Table (1D)  x=front.damper.v m/s  f=front.damper.N N  interp_method=simscape.enum.interpolation.linear  extrap_method=simscape.enum.extrapolation.linear
  instant center : fl_lib/Physical Signals/Lookup Tables/PS Lookup Table (1D)  x=front.z_bp m  f=tan(front.IC_alpha)  interp_method=simscape.enum.interpolation.linear  extrap_method=simscape.enum.extrapolation.linear
  motion ratio : fl_lib/Physical Signals/Lookup Tables/PS Lookup Table (1D)  x=front.z_bp m  f=front.spring.mr_bp  interp_method=simscape.enum.interpolation.linear  extrap_method=simscape.enum.extrapolation.nearest
  pitch center : fl_lib/Physical Signals/Lookup Tables/PS Lookup Table (1D)  x=front.z_bp m  f=tan(-front.PC_alpha)  interp_method=simscape.enum.interpolation.linear  extrap_method=simscape.enum.extrapolation.linear
  spring : fl_lib/Physical Signals/Lookup Tables/PS Lookup Table (1D)  x=front.spring.l m  f=front.spring.N N  interp_method=simscape.enum.interpolation.linear  extrap_method=simscape.enum.extrapolation.linear
  spring1 : fl_lib/Physical Signals/Lookup Tables/PS Lookup Table (1D)  x=front.spring.N(2:end) N  f=front.spring.l(2:end) m  interp_method=simscape.enum.interpolation.linear  extrap_method=simscape.enum.extrapolation.linear
  to camber : fl_lib/Physical Signals/Lookup Tables/PS Lookup Table (2D)  x1=front.tierod_bp m  x2=front.z_bp m  f=front.right.camber_bp rad  interp_method=simscape.enum.interpolation.linear  extrap_method=simscape.enum.extrapolation.linear
  to caster : fl_lib/Physical Signals/Lookup Tables/PS Lookup Table (2D)  x1=front.tierod_bp m  x2=front.z_bp m  f=front.right.caster_bp rad  interp_method=simscape.enum.interpolation.linear  extrap_method=simscape.enum.extrapolation.linear
  to toe : fl_lib/Physical Signals/Lookup Tables/PS Lookup Table (2D)  x1=front.tierod_bp m  x2=front.z_bp m  f=front.right.toe_bp rad  interp_method=simscape.enum.interpolation.linear  extrap_method=simscape.enum.extrapolation.linear
  to x : fl_lib/Physical Signals/Lookup Tables/PS Lookup Table (2D)  x1=front.tierod_bp m  x2=front.z_bp m  f=front.right.x_bp m  interp_method=simscape.enum.interpolation.linear  extrap_method=simscape.enum.extrapolation.linear
  to y : fl_lib/Physical Signals/Lookup Tables/PS Lookup Table (2D)  x1=front.tierod_bp m  x2=front.z_bp m  f=front.right.y_bp m  interp_method=simscape.enum.interpolation.linear  extrap_method=simscape.enum.extrapolation.linear
  pz : PMIOPort  Side=Left
  ARB : PMIOPort  Port=2  Side=Left
  steering : PMIOPort  Port=3  Side=Left
  front : PMIOPort  Port=4  Side=Left
  WC : PMIOPort  Port=5  Side=Right
  meas : Outport
  wires:
  Subsystem1/1(meas) -> meas/1
  From/1 -> Subsystem1/1(damper)
  PS-Simulink Converter/1 -> [B]
  Gain5/1 -> Bus Creator1/2  "FSpring"
  Add/1 -> Bus Creator1/7  "LDamper"
  PS-Simulink Converter6/1 -> [D]
  [D] -> Gain3/1  "FDamper"
  PS-Simulink Converter10/1 -> [F]
  Constant/1 -> Add/2
  [F] -> Gain4/1  "F"
  Gain2/1 -> Bus Creator1/4  "vDamper"
  [C] -> Gain2/1  "vDamper"
  [B] -> Gain1/1, Gain6/1, Add/1  "xDamper"
  [E] -> Gain5/1  "FSpring"
  Bus Creator1/1 -> Goto/1  "damper"
  PS-Simulink Converter7/1 -> [E]
  Gain1/1 -> Bus Creator1/6  "xSpring"
  PS-Simulink Converter5/1 -> [C]
  Gain3/1 -> Bus Creator1/3  "FDamper"
  Gain4/1 -> Bus Creator1/1  "F"
  Gain6/1 -> Bus Creator1/5  "xDamper"
  connections:
  Subsystem1/RConn1 -- Bushing Joint4/RConn1 -- WC/RConn1 -- Inertia1/RConn1 -- FR/RConn1
  front/RConn1 -- Rigid Transform1/LConn1
  Rigid Transform1/RConn1 -- FR1/RConn1 -- Rigid Transform2/LConn1 -- Subsystem1/LConn1
  Bushing Joint4/RConn2 -- pz/RConn1 -- PS Transfer Function1/LConn1
  PS Transfer Function1/RConn1 -- to toe/LConn2 -- to caster/LConn2 -- to camber/LConn2 -- to y/LConn2 -- instant center/LConn1 -- pitch center/LConn1 -- to x/LConn2
  to toe/LConn1 -- steering/RConn1 -- to caster/LConn1 -- to camber/LConn1 -- to x/LConn1 -- to y/LConn1
  Bushing Joint4/RConn3 -- PS Gain2/LConn1
  PS Transfer Function2/RConn1 -- PS Selector/LConn1 -- PS Selector1/LConn1
  PS Product1/RConn1 -- PS Add5/LConn2
  PS Selector1/RConn1 -- PS Product1/LConn2
  PS Selector/RConn1 -- PS Product/LConn2
  PS Add4/RConn1 -- PS Add/LConn1
  instant center/RConn1 -- PS Product1/LConn1
  to camber/RConn1 -- Bushing Joint4/LConn5
  ARB/RConn1 -- PS Add/LConn2
  pitch center/RConn1 -- PS Product/LConn1
  PS Add5/RConn1 -- PS Gain/LConn1
  to y/RConn1 -- Bushing Joint4/LConn3
  PS Gain/RConn1 -- PS Add4/LConn1
  PS Add5/LConn1 -- PS Product/RConn1
  to toe/RConn1 -- Bushing Joint4/LConn7
  to x/RConn1 -- Bushing Joint4/LConn2
  PS Transfer Function2/LConn1 -- Bushing Joint4/RConn4
  PS Add/RConn1 -- Bushing Joint4/LConn4
  to caster/RConn1 -- Bushing Joint4/LConn6
  Bushing Joint4/LConn1 -- Rigid Transform2/RConn1
  PS Divide4/LConn1 -- PS Gain2/RConn1 -- PS Integrator1/LConn1
  damper/LConn1 -- PS Divide4/RConn1 -- PS-Simulink Converter5/LConn1
  PS-Simulink Converter7/LConn1 -- PS Add1/LConn2 -- spring/RConn1
  motion ratio/RConn1 -- PS Divide5/LConn2 -- PS Divide4/LConn2 -- PS Divide3/LConn2
  PS Add1/RConn1 -- PS Divide5/LConn1 -- PS-Simulink Converter10/LConn1
  PS Add7/RConn1 -- PS-Simulink Converter/LConn1 -- spring/LConn1
  PS Divide3/LConn1 -- PS Integrator1/RConn1 -- motion ratio/LConn1
  damper/RConn1 -- PS Add1/LConn1 -- PS-Simulink Converter6/LConn1
  PS Gain1/LConn1 -- PS Divide5/RConn1
  PS Add4/LConn2 -- PS Gain1/RConn1
  spring1/RConn1 -- PS Add7/LConn1
  PS Add7/LConn2 -- PS Divide3/RConn1
  spring1/LConn1 -- PS Constant2/RConn1
